simulink model "Loops8"  (Simulink 8.7)
settings: Solver=ode45  StartTime=0.0  StopTime=10.0  RelTol=1e-3
settings Model: Creator=scaife  LastModifiedBy=bourbouh  ExtModeAutoUpdateStatusClock=off
settings DataIOCC: SignalLoggingSaveFormat=ModelDataLogs  SignalLoggingName=sigsOut
settings OptimizationCC: InitFltsAndDblsToZero=on
settings DebuggingCC: SaveWithParameterizedLinksMsg=none  SignalResolutionControl=TryResolveAllWithWarning  MultiTaskDSMMsg=warning  MultiTaskCondExecSysMsg=none
settings HardwareCC: TargetUnknown=on
settings SFSimCC: SimParseCustomCode=off
settings GRTTargetCC: TargetFcnLib=ansi_tfl_tmw.mat  ModelReferenceCompliant=off  GeneratePreprocessorConditionals=Use local settings  CombineOutputUpdateFcns=off  MatFileLogging=off  GRTInterface=on

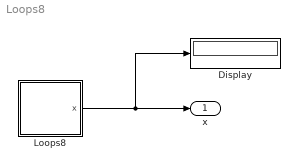
== system Loops8 ==
  Display : Display
  Loops8 : Stateflow chart  TreatAsAtomicUnit=on
  x : Outport
  wires:
  Loops8/1(x) -> Display/1, x/1

== stateflow chart Loops8 ==
  state A
  state B
  state C
  state D
  (default) -> A
  (junction 9) -> C [order 1] : [x==1]
  C -> (junction 9) : {x=2}
  (junction 8) -> A [order 3]
  A -> (junction 8) : {x=0}
  (junction 8) -> (junction 9) [order 1] : [x==0]
  (junction 9) -> (junction 8) [order 3]
  (junction 10) -> (junction 8) [order 3]
  (junction 8) -> (junction 10) [order 2] : [x==2]
  (junction 9) -> (junction 11) [order 2] : [x==0]
  (junction 11) -> (junction 9) [order 3]
  (junction 10) -> (junction 11) [order 1] : [x==1||x==2]
  (junction 11) -> (junction 10) [order 2] : [x==0||x==3]
  (junction 10) -> B [order 2] : [x==0]
  (junction 11) -> D [order 1] : [x==2]
  B -> (junction 10) : {x=1}
  D -> (junction 11) : {x=3}
  data: x output int32
